simulink model "HDLOFDMSynched"  (R2024a)
settings: Solver=FixedStepDiscrete  StartTime=0.0  StopTime=stopTime  RelTol=1e-3
values from neighbouring files (symbols this model uses):
  payloadBitsPerSubcarrierIn = payloadBitsPerSubcarrier    [testOFDMSynched.m]
  payloadCyclicPrefixLenIn = payloadCyclicPrefixLen    [testOFDMSynched.m]
  psduSizeLSB = flip(psduSize)    [testOFDMSynched.m]
undefined symbols (not defined in the file or in its folder): CONST
libraries: HDL_ieee_8021513 x9, hdlsllib x8, dspsrcs4 x2, whdlutilities x2
settings Model: DataTypeOverride=Off  Creator=cotti  LastModifiedBy=cotti
settings OptimizationCC: BlockReduction=off  ConditionallyExecuteInputs=off  DefaultParameterBehavior=Inlined  InheritOutputTypeSmallerThanSingle=on
settings DebuggingCC: AlgebraicLoopMsg=error  ArtificialAlgebraicLoopMsg=error  SingleTaskRateTransMsg=error  UnconnectedInputMsg=warning  UnconnectedOutputMsg=warning  UnconnectedLineMsg=warning
settings HardwareCC: ProdBitPerPointer=32  ProdBitPerSizeT=32  ProdBitPerPtrDiffT=32  ProdLargestAtomicFloat=None  ProdIntDivRoundTo=Undefined  ProdEndianess=Unspecified  ProdWordSize=32  ProdHWDeviceType=ASIC/FPGA->ASIC/FPGA  TargetBitPerLong=64  TargetBitPerPointer=64  TargetBitPerSizeT=64  TargetBitPerPtrDiffT=64  TargetLongLongMode=on  TargetIntDivRoundTo=Zero  TargetEndianess=LittleEndian  TargetWordSize=64  TargetHWDeviceType=Custom Processor->MATLAB Host Computer  ProdEqTarget=off

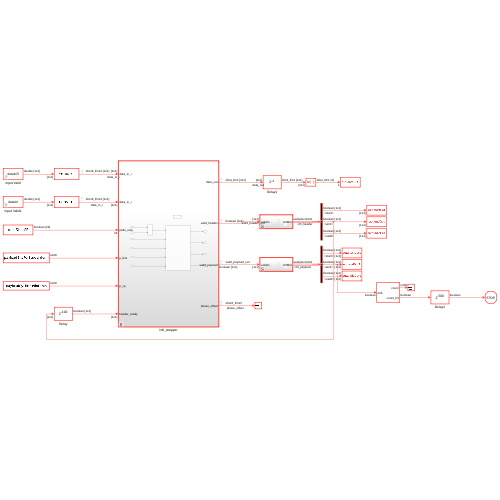
[thumbnail: Simulink's stored preview of the top-level diagram]
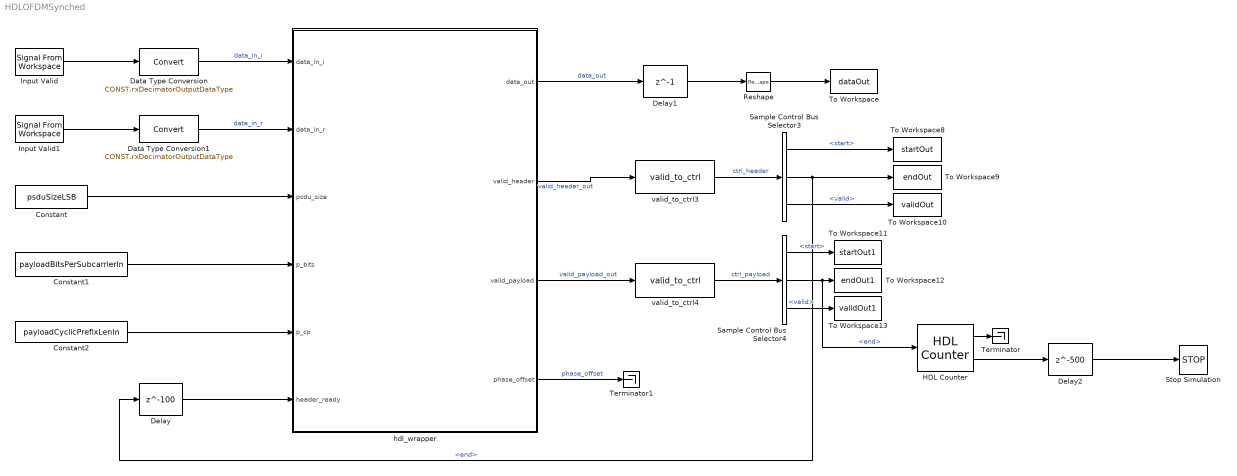
== system HDLOFDMSynched ==
  Constant : Constant  Value=psduSizeLSB  OutDataTypeStr=boolean  SampleTime=-1
  Constant1 : Constant  Value=payloadBitsPerSubcarrierIn  OutDataTypeStr=uint8  SampleTime=-1
  Constant2 : Constant  Value=payloadCyclicPrefixLenIn  OutDataTypeStr=uint8  SampleTime=-1
  Data Type Conversion : DataTypeConversion  OutDataTypeStr=CONST.rxDecimatorOutputDataType  SaturateOnIntegerOverflow=off  RndMeth=Floor
  Data Type Conversion1 : DataTypeConversion  OutDataTypeStr=CONST.rxDecimatorOutputDataType  SaturateOnIntegerOverflow=off  RndMeth=Floor
  Delay : Delay  DelayLength=100  InitialCondition=0  UseCircularBuffer=on
  Delay1 : Delay  DelayLength=1  InitialCondition=0  UseCircularBuffer=on
  Delay2 : Delay  DelayLength=500  InitialCondition=0  UseCircularBuffer=on
  HDL Counter : hdlsllib/Sources/HDL Counter  CountType=Count limited  CountInit=0  CountStep=1  CountMax=totalOFDMSymbols  CountFromType=Initial value  CountFrom=0  CountResetPort=off  CountLoadPort=off  CountEnbPort=on  CountDirPort=off  CountHitOutputPort=on  CountDataType=Unsigned  CountWordLen=8  CountFracLen=0  CountSampTime=1
  Input Valid : dspsrcs4/Signal From Workspace  X=dataInR  Ts=1/CONST.fPHY  nsamps=1  OutputAfterFinalValue=Setting to zero  ignoreOrWarnInputAndFrameLengths=off  OutputFrames=off
  Input Valid1 : dspsrcs4/Signal From Workspace  X=dataInI  Ts=1/CONST.fPHY  nsamps=1  OutputAfterFinalValue=Setting to zero  ignoreOrWarnInputAndFrameLengths=off  OutputFrames=off
  Reshape : Reshape
  Sample Control Bus Selector3 : whdlutilities/Sample Control Bus Selector  OutputSignals=start,end,valid
  Sample Control Bus Selector4 : whdlutilities/Sample Control Bus Selector  OutputSignals=start,end,valid
  Stop Simulation : Stop
  Terminator : Terminator
  Terminator1 : Terminator
  To Workspace : ToWorkspace  VariableName=dataOut  SampleTime=1/CONST.fPHY
      settings: Save2DSignal=2-D array (concatenate along first dimension)
  To Workspace10 : ToWorkspace  VariableName=validOut  SampleTime=1/CONST.fPHY
      settings: Save2DSignal=2-D array (concatenate along first dimension)
  To Workspace11 : ToWorkspace  VariableName=startOut1  SampleTime=1/CONST.fPHY
      settings: Save2DSignal=2-D array (concatenate along first dimension)
  To Workspace12 : ToWorkspace  VariableName=endOut1  SampleTime=1/CONST.fPHY
      settings: Save2DSignal=2-D array (concatenate along first dimension)
  To Workspace13 : ToWorkspace  VariableName=validOut1  SampleTime=1/CONST.fPHY
      settings: Save2DSignal=2-D array (concatenate along first dimension)
  To Workspace8 : ToWorkspace  VariableName=startOut  SampleTime=1/CONST.fPHY
      settings: Save2DSignal=2-D array (concatenate along first dimension)
  To Workspace9 : ToWorkspace  VariableName=endOut  SampleTime=1/CONST.fPHY
      settings: Save2DSignal=2-D array (concatenate along first dimension)
  hdl_wrapper : Subsystem  TreatAsAtomicUnit=on
  valid_to_ctrl3 : HDL_ieee_8021513/valid_to_ctrl  SystemSampleTime=-1  VariantActivationTime=update diagram  AllowFlexibleInterface=on  Latency=0  AutoFrameSizeCalculation=off
      settings: SourceProductName=HDL IEEE 8021513
  valid_to_ctrl4 : HDL_ieee_8021513/valid_to_ctrl  SystemSampleTime=-1  VariantActivationTime=update diagram  AllowFlexibleInterface=on  Latency=0  AutoFrameSizeCalculation=off
      settings: SourceProductName=HDL IEEE 8021513
  wires:
  Input Valid1/1 -> Data Type Conversion1/1
  Input Valid/1 -> Data Type Conversion/1
  HDL Counter/2 -> Delay2/1
  Sample Control Bus Selector3/3 -> To Workspace10/1  "<valid>"
  HDL Counter/1 -> Terminator/1
  valid_to_ctrl4/1 -> Sample Control Bus Selector4/1  "ctrl_payload"
  hdl_wrapper/2(valid_header) -> valid_to_ctrl3/1  "valid_header_out"
  Delay2/1 -> Stop Simulation/1
  Sample Control Bus Selector3/2 -> Delay/1, To Workspace9/1  "<end>"
  Sample Control Bus Selector3/1 -> To Workspace8/1  "<start>"
  Delay1/1 -> Reshape/1
  hdl_wrapper/1(data_out) -> Delay1/1  "data_out"
  Reshape/1 -> To Workspace/1
  Sample Control Bus Selector4/1 -> To Workspace11/1  "<start>"
  Sample Control Bus Selector4/3 -> To Workspace13/1  "<valid>"
  Sample Control Bus Selector4/2 -> HDL Counter/1, To Workspace12/1  "<end>"
  valid_to_ctrl3/1 -> Sample Control Bus Selector3/1  "ctrl_header"
  hdl_wrapper/3(valid_payload) -> valid_to_ctrl4/1  "valid_payload_out"
  Data Type Conversion/1 -> hdl_wrapper/1(data_in_i)  "data_in_i"
  Data Type Conversion1/1 -> hdl_wrapper/2(data_in_r)  "data_in_r"
  hdl_wrapper/4(phase_offset) -> Terminator1/1  "phase_offset"
  Constant/1 -> hdl_wrapper/3(psdu_size)
  Constant1/1 -> hdl_wrapper/4(p_bits)
  Constant2/1 -> hdl_wrapper/5(p_cp)
  Delay/1 -> hdl_wrapper/6(header_ready)

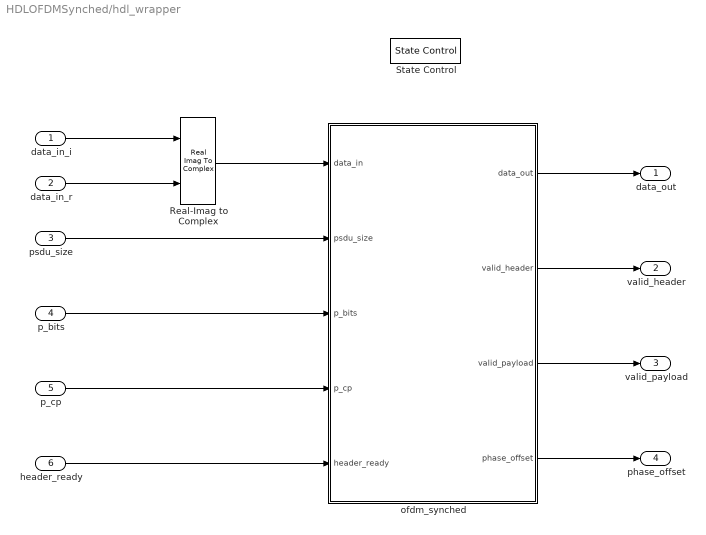
== system HDLOFDMSynched/hdl_wrapper ==
  data_in_i : Inport
  data_in_r : Inport  Port=2
  psdu_size : Inport  Port=3
  p_bits : Inport  Port=4
  p_cp : Inport  Port=5
  header_ready : Inport  Port=6
  Real-Imag to Complex : RealImagToComplex
  State Control : StateControl  StateControl=Synchronous
  ofdm_synched : Subsystem
  data_out : Outport  VectorParamsAs1DForOutWhenUnconnected=off
  valid_header : Outport  Port=2  VectorParamsAs1DForOutWhenUnconnected=off
  valid_payload : Outport  Port=3  VectorParamsAs1DForOutWhenUnconnected=off
  phase_offset : Outport  Port=4  VectorParamsAs1DForOutWhenUnconnected=off
  wires:
  ofdm_synched/2(valid_header) -> valid_header/1
  ofdm_synched/3(valid_payload) -> valid_payload/1
  data_in_r/1 -> Real-Imag to Complex/2
  ofdm_synched/1(data_out) -> data_out/1
  Real-Imag to Complex/1 -> ofdm_synched/1(data_in)
  data_in_i/1 -> Real-Imag to Complex/1
  psdu_size/1 -> ofdm_synched/2(psdu_size)
  p_bits/1 -> ofdm_synched/3(p_bits)
  p_cp/1 -> ofdm_synched/4(p_cp)
  ofdm_synched/4(phase_offset) -> phase_offset/1
  header_ready/1 -> ofdm_synched/5(header_ready)

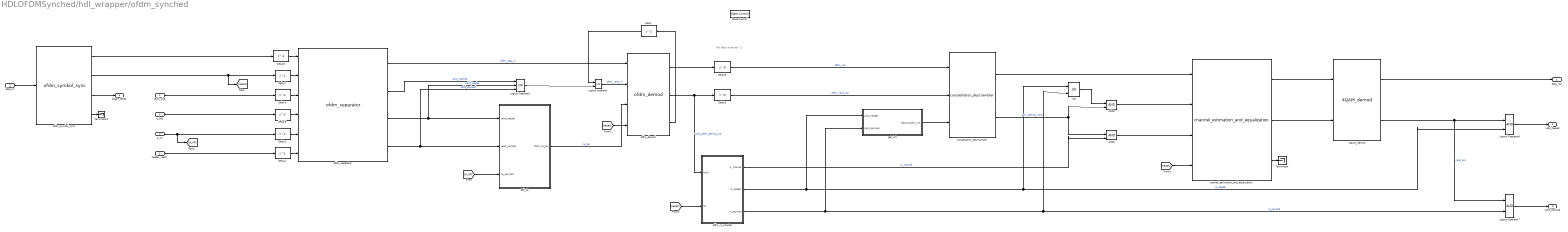
== system HDLOFDMSynched/hdl_wrapper/ofdm_synched ==
  note: This delay must be > 2
  data_in : Inport
  psdu_size : Inport  Port=2
  p_bits : Inport  Port=3
  p_cp : Inport  Port=4
  header_ready : Inport  Port=5
  4QAM_demod : HDL_ieee_8021513/4QAM_demod  SystemSampleTime=-1  VariantActivationTime=update diagram  AllowFlexibleInterface=on  Latency=0  AutoFrameSizeCalculation=off
      settings: SourceProductName=HDL IEEE 8021513
  AND1 : Logic  IconShape=distinctive  AllPortsSameDT=off  OutDataTypeStr=boolean
  AND2 : Logic  IconShape=distinctive  AllPortsSameDT=off  OutDataTypeStr=boolean
  Delay{,1..4,7..8} (7 alike) : Delay  DelayLength=1  InitialCondition=0  UseCircularBuffer=on
  Delay5 : Delay  DelayLength=5  InitialCondition=0  UseCircularBuffer=on
  Delay6 : Delay  DelayLength=5  InitialCondition=0  UseCircularBuffer=on
  Logical Operator : Logic  IconShape=distinctive  AllPortsSameDT=off  OutDataTypeStr=boolean
  Logical Operator1 : Logic  Operator=OR  Inputs=3  IconShape=distinctive  AllPortsSameDT=off  OutDataTypeStr=boolean
  Logical Operator6 : Logic  IconShape=distinctive  AllPortsSameDT=off  OutDataTypeStr=boolean
  Logical Operator7 : Logic  IconShape=distinctive  AllPortsSameDT=off  OutDataTypeStr=boolean
  OR : Logic  Operator=OR  IconShape=distinctive  AllPortsSameDT=off  OutDataTypeStr=boolean
  State Control : StateControl  StateControl=Synchronous
  Terminator : Terminator
  Terminator1 : Terminator
  channel_estimation_and_equalization : HDL_ieee_8021513/channel_estimation_and_equalization  SystemSampleTime=-1  VariantActivationTime=update diagram  AllowFlexibleInterface=on  Latency=0  AutoFrameSizeCalculation=off
      settings: SourceProductName=HDL IEEE 8021513
  constellation_descrambler : HDL_ieee_8021513/constellation_descrambler  SystemSampleTime=-1  VariantActivationTime=update diagram  AllowFlexibleInterface=on  Latency=0  AutoFrameSizeCalculation=off
      settings: SourceProductName=HDL IEEE 8021513
  get_cp : Subsystem
  get_init : Subsystem
  ofdm_demod : HDL_ieee_8021513/ofdm_demod  SystemSampleTime=-1  VariantActivationTime=update diagram  AllowFlexibleInterface=on  Latency=0  AutoFrameSizeCalculation=off
      settings: SourceProductName=HDL IEEE 8021513
  ofdm_rx_counter : Subsystem
  ofdm_separator : HDL_ieee_8021513/ofdm_separator  SystemSampleTime=-1  VariantActivationTime=update diagram  AllowFlexibleInterface=on  Latency=0  AutoFrameSizeCalculation=off
      settings: SourceProductName=HDL IEEE 8021513
  ofdm_symbol_sync : HDL_ieee_8021513/ofdm_symbol_sync  SystemSampleTime=-1  VariantActivationTime=update diagram  AllowFlexibleInterface=on  Latency=0  AutoFrameSizeCalculation=off
      settings: SourceProductName=HDL IEEE 8021513
  data_out : Outport  VectorParamsAs1DForOutWhenUnconnected=off
  valid_header : Outport  Port=2  VectorParamsAs1DForOutWhenUnconnected=off
  valid_payload : Outport  Port=3  VectorParamsAs1DForOutWhenUnconnected=off
  phase_offset : Outport  Port=4  VectorParamsAs1DForOutWhenUnconnected=off
  wires:
  Delay3/1 -> ofdm_separator/4
  channel_estimation_and_equalization/3 -> Terminator/1
  OR/1 -> AND2/1
  ofdm_separator/1 -> ofdm_demod/1  "ofdm_data_in"
  channel_estimation_and_equalization/1 -> 4QAM_demod/1
  p_bits/1 -> Delay3/1
  constellation_descrambler/1 -> channel_estimation_and_equalization/1
  AND1/1 -> channel_estimation_and_equalization/3
  4QAM_demod/1 -> data_out/1
  ofdm_rx_counter/2(is_header) -> Logical Operator6/2, OR/1, get_init/1(valid_header)  "is_header"
  ofdm_separator/2 -> Logical Operator1/1  "valid_channel"
  Delay5/1 -> constellation_descrambler/2  "ofdm_valid_out"
  [p_cp] -> get_cp/3(cp_payload)
  [reset] -> ofdm_demod/4
  p_cp/1 -> [p_cp], Delay2/1
  get_cp/1(ofdm_cp_len) -> ofdm_demod/3  "cp_len"
  4QAM_demod/2 -> Logical Operator6/1, Logical Operator7/1  "valid_out"
  Delay2/1 -> ofdm_separator/5
  Logical Operator/1 -> ofdm_demod/2  "ofdm_valid_in"
  Delay7/1 -> ofdm_separator/2
  Logical Operator6/1 -> valid_header/1
  ofdm_demod/3 -> Delay/1
  psdu_size/1 -> Delay4/1
  Logical Operator1/1 -> Logical Operator/2
  ofdm_rx_counter/3(is_payload) -> Logical Operator7/2, OR/2, get_init/2(valid_payload)  "is_payload"
  get_init/1(descrambler_init) -> constellation_descrambler/3
  Delay/1 -> Logical Operator/1
  Delay8/1 -> ofdm_separator/1
  Delay4/1 -> ofdm_separator/3
  AND2/1 -> channel_estimation_and_equalization/2
  ofdm_rx_counter/1(is_channel) -> AND1/2  "is_channel"
  [reset] -> ofdm_rx_counter/2(rst)
  header_ready/1 -> Delay1/1
  channel_estimation_and_equalization/2 -> 4QAM_demod/2
  Delay6/1 -> constellation_descrambler/1  "ofdm_out"
  [reset] -> channel_estimation_and_equalization/4
  ofdm_separator/3 -> Logical Operator1/2, get_cp/1(valid_header)  "valid_header"
  ofdm_demod/2 -> ofdm_rx_counter/1(valid), Delay5/1  "valid_ofdm_demod_out"
  Logical Operator7/1 -> valid_payload/1
  ofdm_demod/1 -> Delay6/1
  ofdm_separator/4 -> get_cp/2(valid_payload), Logical Operator1/3  "valid_payload"
  Delay1/1 -> ofdm_separator/6
  constellation_descrambler/2 -> AND1/1, AND2/2  "qam_demod_valid"
  data_in/1 -> ofdm_symbol_sync/1
  ofdm_symbol_sync/2 -> Delay7/1, [reset]
  ofdm_symbol_sync/1 -> Delay8/1
  ofdm_symbol_sync/4 -> Terminator1/1
  ofdm_symbol_sync/3 -> phase_offset/1

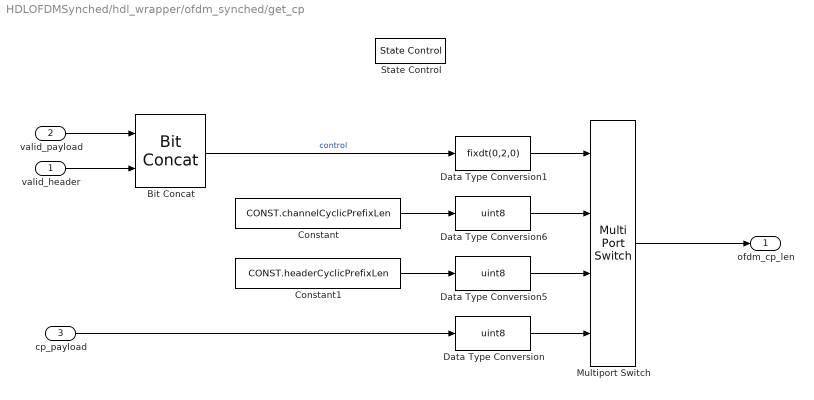
== system HDLOFDMSynched/hdl_wrapper/ofdm_synched/get_cp ==
  valid_header : Inport
  valid_payload : Inport  Port=2
  cp_payload : Inport  Port=3
  Bit Concat : hdlsllib/Logic and Bit Operations/Bit Concat  numInputs=2
  Constant : Constant  Value=CONST.channelCyclicPrefixLen  OutDataTypeStr=uint8  SampleTime=-1
  Constant1 : Constant  Value=CONST.headerCyclicPrefixLen  OutDataTypeStr=uint8  SampleTime=-1
  Data Type Conversion : DataTypeConversion  OutDataTypeStr=uint8  SaturateOnIntegerOverflow=off  RndMeth=Floor
  Data Type Conversion1 : DataTypeConversion  OutDataTypeStr=fixdt(0,2,0)  SaturateOnIntegerOverflow=off  RndMeth=Floor
  Data Type Conversion5 : DataTypeConversion  OutDataTypeStr=uint8  SaturateOnIntegerOverflow=off  RndMeth=Floor
  Data Type Conversion6 : DataTypeConversion  OutDataTypeStr=uint8  SaturateOnIntegerOverflow=off  RndMeth=Floor
  Multiport Switch : MultiPortSwitch  DataPortOrder=Zero-based contiguous  zeroidx=on  SaturateOnIntegerOverflow=off
  State Control : StateControl  StateControl=Synchronous
  ofdm_cp_len : Outport
  wires:
  Data Type Conversion1/1 -> Multiport Switch/1
  valid_header/1 -> Bit Concat/2
  valid_payload/1 -> Bit Concat/1
  Data Type Conversion/1 -> Multiport Switch/4
  Data Type Conversion5/1 -> Multiport Switch/3
  Data Type Conversion6/1 -> Multiport Switch/2
  Multiport Switch/1 -> ofdm_cp_len/1
  cp_payload/1 -> Data Type Conversion/1
  Constant/1 -> Data Type Conversion6/1
  Constant1/1 -> Data Type Conversion5/1
  Bit Concat/1 -> Data Type Conversion1/1  "control"

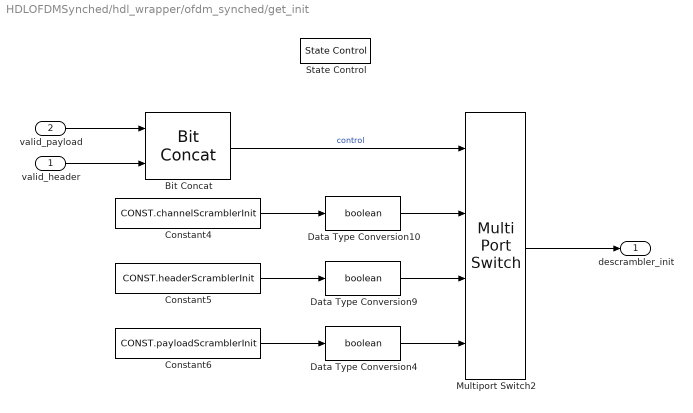
== system HDLOFDMSynched/hdl_wrapper/ofdm_synched/get_init ==
  valid_header : Inport
  valid_payload : Inport  Port=2
  Bit Concat : hdlsllib/Logic and Bit Operations/Bit Concat  numInputs=2
  Constant4 : Constant  Value=CONST.channelScramblerInit  OutDataTypeStr=uint8  SampleTime=-1
  Constant5 : Constant  Value=CONST.headerScramblerInit  OutDataTypeStr=uint8  SampleTime=-1
  Constant6 : Constant  Value=CONST.payloadScramblerInit  OutDataTypeStr=uint8  SampleTime=-1
  Data Type Conversion10 : DataTypeConversion  OutDataTypeStr=boolean  SaturateOnIntegerOverflow=off  RndMeth=Floor
  Data Type Conversion4 : DataTypeConversion  OutDataTypeStr=boolean  SaturateOnIntegerOverflow=off  RndMeth=Floor
  Data Type Conversion9 : DataTypeConversion  OutDataTypeStr=boolean  SaturateOnIntegerOverflow=off  RndMeth=Floor
  Multiport Switch2 : MultiPortSwitch  DataPortOrder=Zero-based contiguous  zeroidx=on  SaturateOnIntegerOverflow=off  InputSameDT=off
  State Control : StateControl  StateControl=Synchronous
  descrambler_init : Outport
  wires:
  Bit Concat/1 -> Multiport Switch2/1  "control"
  valid_header/1 -> Bit Concat/2
  valid_payload/1 -> Bit Concat/1
  Data Type Conversion10/1 -> Multiport Switch2/2
  Multiport Switch2/1 -> descrambler_init/1
  Constant4/1 -> Data Type Conversion10/1
  Constant5/1 -> Data Type Conversion9/1
  Data Type Conversion4/1 -> Multiport Switch2/4
  Constant6/1 -> Data Type Conversion4/1
  Data Type Conversion9/1 -> Multiport Switch2/3

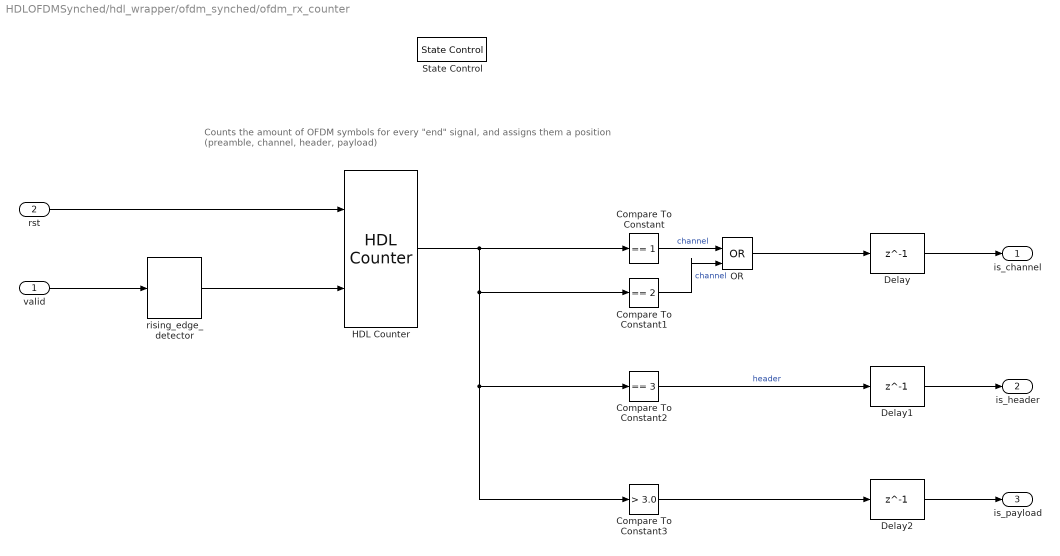
== system HDLOFDMSynched/hdl_wrapper/ofdm_synched/ofdm_rx_counter ==
  note: Counts the amount of OFDM symbols for every "end" signal, and assigns them a position (preamble, channel, header, payload)
  valid : Inport
  rst : Inport  Port=2
  Compare To Constant : hdlsllib/Logic and Bit Operations/Compare To Constant  relop===  const=1  OutDataTypeStr=boolean
  Compare To Constant1 : hdlsllib/Logic and Bit Operations/Compare To Constant  relop===  const=2  OutDataTypeStr=boolean
  Compare To Constant2 : hdlsllib/Logic and Bit Operations/Compare To Constant  relop===  const=3  OutDataTypeStr=boolean
  Compare To Constant3 : hdlsllib/Logic and Bit Operations/Compare To Constant  relop=>  const=3.0  OutDataTypeStr=boolean
  Delay : Delay  DelayLength=1  InitialCondition=0  UseCircularBuffer=on
  Delay1 : Delay  DelayLength=1  InitialCondition=0  UseCircularBuffer=on
  Delay2 : Delay  DelayLength=1  InitialCondition=0  UseCircularBuffer=on
  HDL Counter : hdlsllib/Sources/HDL Counter  CountType=Free running  CountInit=0  CountStep=1  CountMax=25  CountFromType=Initial value  CountFrom=0  CountResetPort=on  CountLoadPort=off  CountEnbPort=on  CountDirPort=off  CountHitOutputPort=off  CountDataType=Unsigned  CountWordLen=16  CountFracLen=0  CountSampTime=1
  OR : Logic  Operator=OR  IconShape=distinctive  AllPortsSameDT=off  OutDataTypeStr=boolean
  State Control : StateControl  StateControl=Synchronous
  rising_edge_detector : HDL_ieee_8021513/rising_edge_detector  SystemSampleTime=-1  VariantActivationTime=update diagram  AllowFlexibleInterface=on  Latency=0  AutoFrameSizeCalculation=off
      settings: SourceProductName=HDL IEEE 8021513
  is_channel : Outport
  is_header : Outport  Port=2
  is_payload : Outport  Port=3
  wires:
  valid/1 -> rising_edge_detector/1
  rising_edge_detector/1 -> HDL Counter/2
  HDL Counter/1 -> Compare To Constant/1, Compare To Constant3/1, Compare To Constant2/1, Compare To Constant1/1
  Compare To Constant2/1 -> Delay1/1  "header"
  rst/1 -> HDL Counter/1
  OR/1 -> Delay/1
  Compare To Constant/1 -> OR/1  "channel"
  Compare To Constant1/1 -> OR/2  "channel"
  Compare To Constant3/1 -> Delay2/1
  Delay/1 -> is_channel/1
  Delay1/1 -> is_header/1
  Delay2/1 -> is_payload/1
